simulink model "hw4_step"  (R2018b)
settings: Solver=VariableStepAuto  StartTime=0.0  StopTime=2  RelTol=1e-3
values from neighbouring files (symbols this model uses):
  A = [0 1;b 0]    [loadpars.m]    (also in loadpars_stbl_unstbl_pts.m; reg_attract_hw.m)
  B = [0;a]    [loadpars.m]    (also in loadpars_stbl_unstbl_pts.m; reg_attract_hw.m)
  dx0 = [0;0]    [loadpars.m]    (also in loadpars_stbl_unstbl_pts.m = [0.001;0])
  K = lqr(A,B,Q,R)    [loadpars.m]    (also in loadpars_stbl_unstbl_pts.m; reg_attract_hw.m)
  ueq = ieq    [loadpars.m]    (also in loadpars_stbl_unstbl_pts.m; reg_attract_hw.m)
  x0 = xeq+dx0    [loadpars.m]    (also in loadpars_stbl_unstbl_pts.m = [xi(1,1);yi(1,1)])
  xeq = [xeq1;xeq2]    [loadpars.m]    (also in loadpars_stbl_unstbl_pts.m; reg_attract_hw.m)
undefined symbols (not defined in the file or in its folder): stateder
settings Model: Creator=rhanz  LastModifiedBy=arsh
settings SFSimCC: SimUseLocalCustomCode=off
settings RTWCC: RTWUseLocalCustomCode=off
settings CodeAppCC: StateflowObjectComments=on

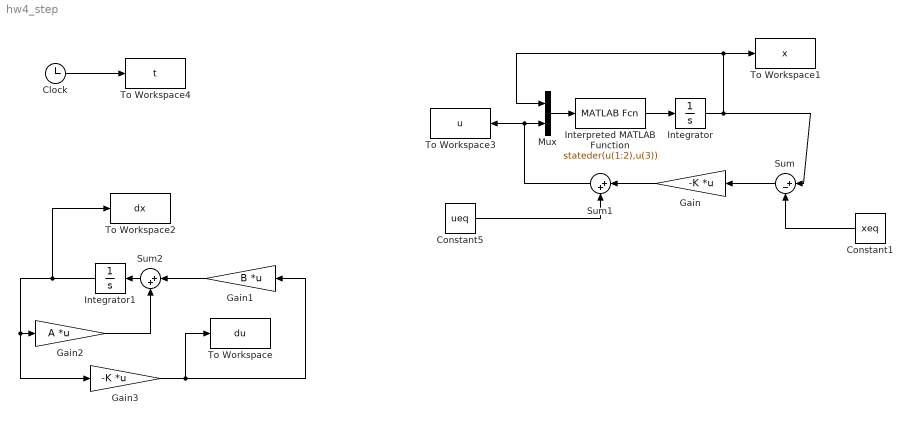
== system hw4_step ==
  Clock : Clock
  Constant1 : Constant  Value=xeq
  Constant5 : Constant  Value=ueq
  Gain : Gain  Gain=-K  Multiplication=Matrix(K*u) (u vector)
  Gain1 : Gain  Gain=B  Multiplication=Matrix(K*u) (u vector)
  Gain2 : Gain  Gain=A  Multiplication=Matrix(K*u) (u vector)
  Gain3 : Gain  Gain=-K  Multiplication=Matrix(K*u) (u vector)
  Integrator : Integrator  InitialCondition=x0
  Integrator1 : Integrator  InitialCondition=dx0
  Interpreted MATLAB Function : MATLABFcn  MATLABFcn=stateder(u(1:2),u(3))
  Mux : Mux  Inputs=2
  Sum : Sum  Inputs=|+-
  Sum1 : Sum  Inputs=|++
  Sum2 : Sum  Inputs=|++
  To Workspace : ToWorkspace  VariableName=du  SampleTime=-1
  To Workspace1 : ToWorkspace  VariableName=x  SampleTime=-1
  To Workspace2 : ToWorkspace  VariableName=dx  SampleTime=-1
  To Workspace3 : ToWorkspace  VariableName=u  SampleTime=-1
  To Workspace4 : ToWorkspace  VariableName=t  SampleTime=-1
  wires:
  Sum2/1 -> Integrator1/1
  Gain1/1 -> Sum2/1
  Gain2/1 -> Sum2/2
  Integrator1/1 -> To Workspace2/1, Gain3/1, Gain2/1
  Clock/1 -> To Workspace4/1
  Gain3/1 -> To Workspace/1, Gain1/1
  Gain/1 -> Sum1/1
  Interpreted MATLAB Function/1 -> Integrator/1
  Mux/1 -> Interpreted MATLAB Function/1
  Sum/1 -> Gain/1
  Integrator/1 -> Sum/1, Mux/1, To Workspace1/1
  Sum1/1 -> Mux/2, To Workspace3/1
  Constant1/1 -> Sum/2
  Constant5/1 -> Sum1/2
